simulink model "s__hover_lqg_1"  (R2025b)
settings: Solver=VariableStepAuto  StartTime=0.0  StopTime=100  RelTol=1e-3
undefined symbols (not defined in the file): A, B, C, K, sysKF
settings Model: Creator=admin  LastModifiedBy=USER_NAME
settings SolverCC: AlgebraicLoopSolver=TrustRegion
settings DataIOCC: ReturnWorkspaceOutputs=off
settings OptimizationCC: LifeSpan=inf
settings DebuggingCC: UnconnectedInputMsg=warning  UnconnectedOutputMsg=warning  UnconnectedLineMsg=warning  SFExecutionAtInitializationDiag=none  ArithmeticOperatorsInVariantConditions=warning
settings ModelReferenceCC: EnableRefExpFcnMdlSchedulingChecks=on
settings SFSimCC: SimUseLocalCustomCode=off  CustomCodeUndefinedFunction=UseInterfaceOnly
settings RTWCC: RTWUseLocalCustomCode=off  GPUComputeCapability=3.5
settings CodeAppCC: StateflowObjectComments=on

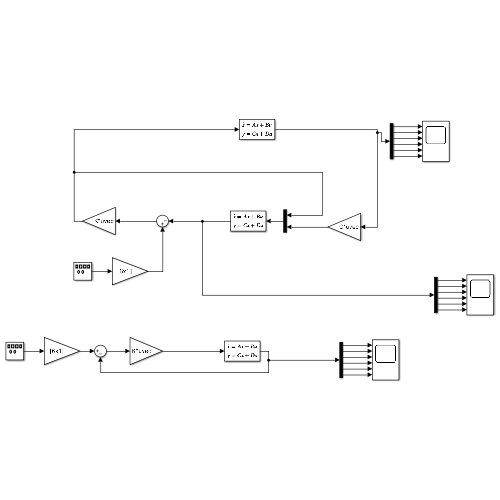
[thumbnail: Simulink's stored preview of the top-level diagram]
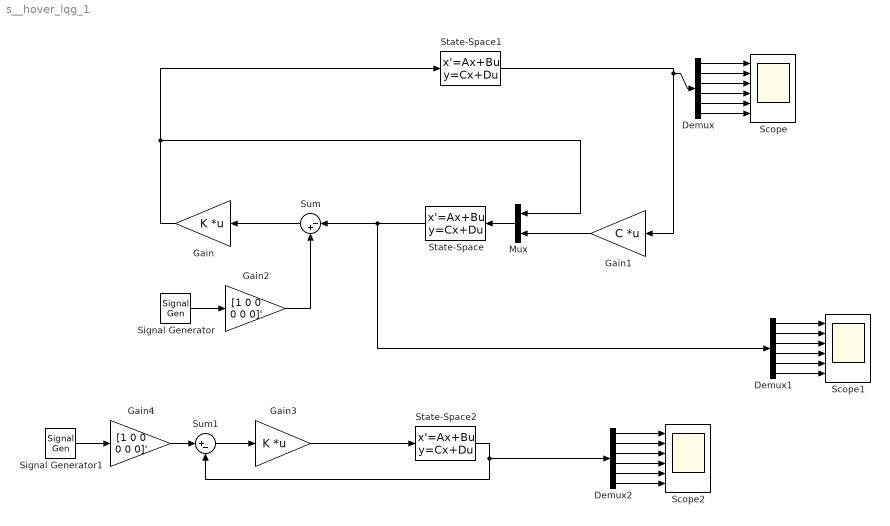
== system s__hover_lqg_1 ==
  Demux : Demux  Outputs=6
  Demux1 : Demux  Outputs=6
  Demux2 : Demux  Outputs=6
  Gain : Gain  Gain=K  Multiplication=Matrix(K*u) (u vector)
  Gain1 : Gain  Gain=C  Multiplication=Matrix(K*u) (u vector)
  Gain2 : Gain  Gain=[1 0 0 0 0 0]'
  Gain3 : Gain  Gain=K  Multiplication=Matrix(K*u) (u vector)
  Gain4 : Gain  Gain=[1 0 0 0 0 0]'
  Mux : Mux  Inputs=2
  Scope : Scope  NumInputPorts=6
      settings: ActiveDisplayYMinimum=-0.98158660717507507  ActiveDisplayYMaximum=0.98056577332498085
  Scope1 : Scope  NumInputPorts=6
      settings: ActiveDisplayYMinimum=-1  ActiveDisplayYMaximum=1
  Scope2 : Scope  NumInputPorts=6
      settings: ActiveDisplayYMinimum=-1  ActiveDisplayYMaximum=1  DataLoggingVariableName=ScopeData2
  Signal Generator : SignalGenerator  WaveForm=square  Units=rad/sec
  Signal Generator1 : SignalGenerator  WaveForm=square  Units=rad/sec
  State-Space : StateSpace  A=sysKF.a  B=sysKF.b  C=sysKF.c  D=sysKF.d  InitialCondition=[0 0 0 0 0 0]
  State-Space1 : StateSpace  A=A  B=B  C=ones(6)  D=zeros(6, 4)  InitialCondition=[0 0 0 0 0 0]
  State-Space2 : StateSpace  A=A  B=B  C=ones(6)  D=zeros(6, 4)  InitialCondition=[0 0 0 0 0 0]
  Sum : Sum  Inputs=|-+
  Sum1 : Sum  Inputs=|+-
  wires:
  State-Space1/1 -> Demux/1, Gain1/1
  Gain/1 -> State-Space1/1, Mux/1
  Gain1/1 -> Mux/2
  Mux/1 -> State-Space/1
  Sum/1 -> Gain/1
  Signal Generator/1 -> Gain2/1
  Demux/1 -> Scope/1
  Demux/2 -> Scope/2
  Demux/3 -> Scope/3
  Demux/4 -> Scope/4
  Demux/5 -> Scope/5
  Demux/6 -> Scope/6
  Gain2/1 -> Sum/2
  Demux1/1 -> Scope1/1
  Demux1/2 -> Scope1/2
  Demux1/3 -> Scope1/3
  Demux1/4 -> Scope1/4
  Demux1/5 -> Scope1/5
  Demux1/6 -> Scope1/6
  State-Space/1 -> Demux1/1, Sum/1
  Gain3/1 -> State-Space2/1
  Gain4/1 -> Sum1/1
  Signal Generator1/1 -> Gain4/1
  State-Space2/1 -> Demux2/1, Sum1/2
  Sum1/1 -> Gain3/1
  Demux2/1 -> Scope2/1
  Demux2/2 -> Scope2/2
  Demux2/3 -> Scope2/3
  Demux2/4 -> Scope2/4
  Demux2/5 -> Scope2/5
  Demux2/6 -> Scope2/6
